simulink subsystem "MLI_20_layer"  (R2024b)
settings: Solver=VariableStepAuto  StartTime=0.0  StopTime=10.0  RelTol=1e-3
settings Model: Creator=MW  LastModifiedBy=MW

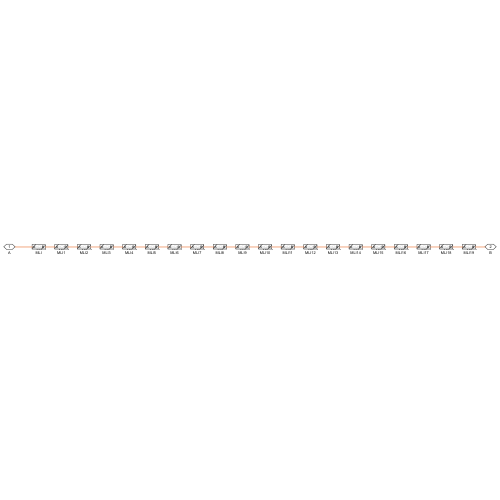
[thumbnail: Simulink's stored preview of the top-level diagram]
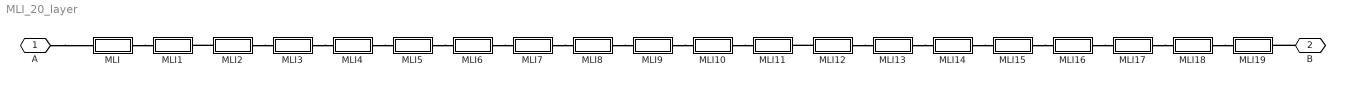
== system MLI_20_layer ==
  MLI{,1..19} (20 alike) : Subsystem  ReferencedSubsystem=MIL_1_layer_radiative
      settings: PortSchema="{\"entries\":[{\"content\":{\"sides\":[{\"content\":{\"connectorIds\":[\"LConn1\"]},\"type\":\"ConnectorPlacement.EquallySpacedRectSide\",\"uuid\":\"13959ff0-7161-4264-b74c-d5f6fc1fc79f\"},{\"content\":{\"connectorIds\":[\"LConn2\"],\"side\":\"RIGHT\"},\"type\":\"ConnectorPlacement.EquallySpacedRectSide\",\"uuid\":\"0144929d-c826-44a3-abc2-3c69c72d534c\"},{\"content\":{\"side\":\"TOP\"},\"type\":\"ConnectorPlacement.EquallySpacedRectSide\",\"uuid\":\"bda55155-c7f6-4e1e-b7ae-8f65907cbe02\"}]},\"type\":\"ConnectorPlacement.EquallySpacedConnector\",\"uuid\":\"e24db636-ea4a-4050-86a0-b249fb595212\"}],\"packageUris\":[\"http://schema.mathworks.com/mf0/Connector/R2020b\"],\"version\":\"1.0\"}"
  A : PMIOPort  Side=Left
  B : PMIOPort  Port=2  Side=Left
  connections:
  MLI16/LConn2 -- MLI17/LConn1
  MLI4/LConn2 -- MLI5/LConn1
  MLI8/LConn2 -- MLI9/LConn1
  MLI13/LConn2 -- MLI14/LConn1
  MLI5/LConn2 -- MLI6/LConn1
  B/RConn1 -- MLI19/LConn2
  MLI2/LConn2 -- MLI3/LConn1
  MLI14/LConn2 -- MLI15/LConn1
  MLI7/LConn2 -- MLI8/LConn1
  MLI3/LConn2 -- MLI4/LConn1
  MLI9/LConn2 -- MLI10/LConn1
  MLI6/LConn2 -- MLI7/LConn1
  MLI17/LConn2 -- MLI18/LConn1
  MLI/LConn2 -- MLI1/LConn1
  MLI12/LConn1 -- MLI11/LConn2
  MLI10/LConn2 -- MLI11/LConn1
  MLI12/LConn2 -- MLI13/LConn1
  MLI2/LConn1 -- MLI1/LConn2
  MLI15/LConn2 -- MLI16/LConn1
  MLI18/LConn2 -- MLI19/LConn1
  A/RConn1 -- MLI/LConn1
